simulink model "C20259_DiegoAlfaro_G01"  (R2023b)
settings: Solver=ode4  StartTime=0.0  StopTime=20  FixedStep=1e-4  RelTol=1e-3
undefined symbols (not defined in the file): kp
libraries: simulink x1
settings Model: Creator=daas0  LastModifiedBy=daas0

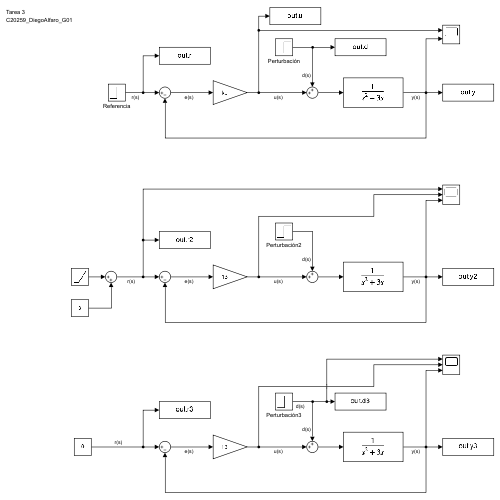
[thumbnail: Simulink's stored preview of the top-level diagram]
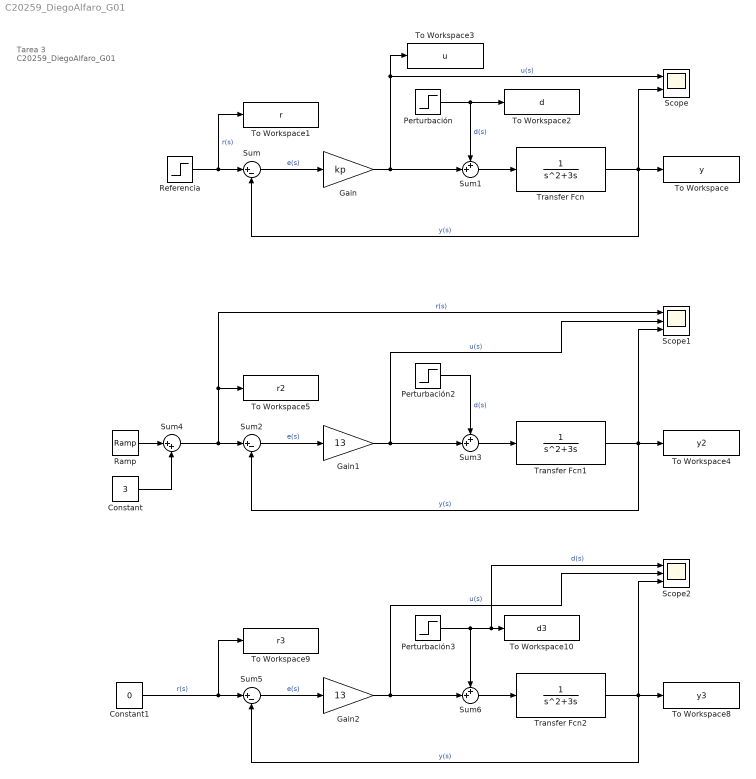
== system C20259_DiegoAlfaro_G01 ==
  note: Tarea 3
      | C20259_DiegoAlfaro_G01
  Constant : Constant  Value=3
  Constant1 : Constant  Value=0
  Gain : Gain  Gain=kp
  Gain1 : Gain  Gain=13
  Gain2 : Gain  Gain=13
  Perturbación : Step  Time=10  After=2  SampleTime=0
  Perturbación2 : Step  Time=10  After=0  SampleTime=0
  Perturbación3 : Step  Time=0  SampleTime=0
  Ramp : simulink/Sources/Ramp  slope=1  start=0  InitialOutput=0
  Referencia : Step  Time=0  After=2  SampleTime=0
  Scope : Scope  NumInputPorts=2
  Scope1 : Scope  NumInputPorts=3
  Scope2 : Scope  NumInputPorts=3
  Sum : Sum  Inputs=|+-
  Sum1 : Sum  Inputs=++|
  Sum2 : Sum  Inputs=|+-
  Sum3 : Sum  Inputs=++|
  Sum4 : Sum  Inputs=|++
  Sum5 : Sum  Inputs=|+-
  Sum6 : Sum  Inputs=++|
  To Workspace : ToWorkspace  VariableName=y  SaveFormat=Timeseries  SampleTime=-1
  To Workspace1 : ToWorkspace  VariableName=r  SaveFormat=Timeseries  SampleTime=-1
  To Workspace10 : ToWorkspace  VariableName=d3  SaveFormat=Timeseries  SampleTime=-1
  To Workspace2 : ToWorkspace  VariableName=d  SaveFormat=Timeseries  SampleTime=-1
  To Workspace3 : ToWorkspace  VariableName=u  SaveFormat=Timeseries  SampleTime=-1
  To Workspace4 : ToWorkspace  VariableName=y2  SaveFormat=Timeseries  SampleTime=-1
  To Workspace5 : ToWorkspace  VariableName=r2  SaveFormat=Timeseries  SampleTime=-1
  To Workspace8 : ToWorkspace  VariableName=y3  SaveFormat=Timeseries  SampleTime=-1
  To Workspace9 : ToWorkspace  VariableName=r3  SaveFormat=Timeseries  SampleTime=-1
  Transfer Fcn : TransferFcn  Denominator=[1 3 0]
  Transfer Fcn1 : TransferFcn  Denominator=[1 3 0]
  Transfer Fcn2 : TransferFcn  Denominator=[1 3 0]
  wires:
  Perturbación/1 -> To Workspace2/1, Sum1/1  "d(s)"
  Gain/1 -> Sum1/2, To Workspace3/1, Scope/1  "u(s)"
  Referencia/1 -> To Workspace1/1, Sum/1  "r(s)"
  Transfer Fcn/1 -> To Workspace/1, Scope/2, Sum/2  "y(s)"
  Sum/1 -> Gain/1  "e(s)"
  Sum1/1 -> Transfer Fcn/1
  Gain1/1 -> Sum3/2, Scope1/2  "u(s)"
  Sum3/1 -> Transfer Fcn1/1
  Sum2/1 -> Gain1/1  "e(s)"
  Transfer Fcn1/1 -> To Workspace4/1, Scope1/3, Sum2/2  "y(s)"
  Perturbación2/1 -> Sum3/1  "d(s)"
  Sum4/1 -> Scope1/1, To Workspace5/1, Sum2/1  "r(s)"
  Ramp/1 -> Sum4/1
  Constant/1 -> Sum4/2
  Perturbación3/1 -> Scope2/1, To Workspace10/1, Sum6/1  "d(s)"
  Sum5/1 -> Gain2/1  "e(s)"
  Gain2/1 -> Sum6/2, Scope2/2  "u(s)"
  Constant1/1 -> To Workspace9/1, Sum5/1  "r(s)"
  Sum6/1 -> Transfer Fcn2/1
  Transfer Fcn2/1 -> To Workspace8/1, Scope2/3, Sum5/2  "y(s)"
